simulink model "HW4_simulink"  (R2017b)
settings: Solver=VariableStepAuto  StartTime=0.0  StopTime=.167  RelTol=1e-3
values from neighbouring files (symbols this model uses):
  B = 0.8    [HW4_code.m]
  ia = 4    [HW4_code.m]
  l = 0.8    [HW4_code.m]
  r = 0.05    [HW4_code.m]
  w = 376.99    [HW4_code.m]
settings Model: Creator=Andrew McCullough  LastModifiedBy=Andrew McCullough

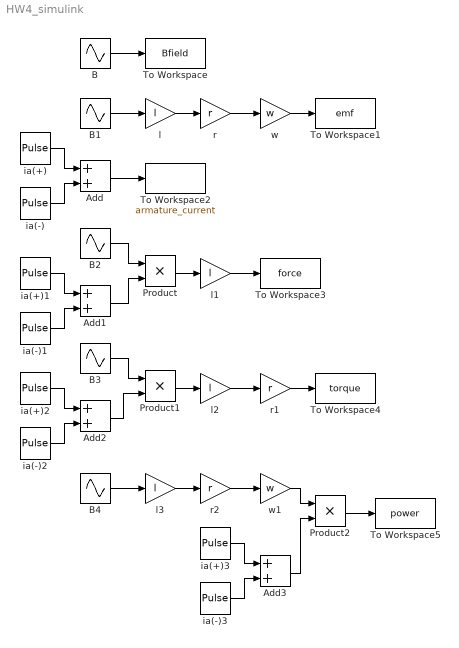
== system HW4_simulink ==
  Add{,1..3} (4 alike) : Sum
  B{,1..4} (5 alike) : Sin  Amplitude=B  Frequency=w  Phase=pi/2  SampleTime=.00001
  Product : Product
  Product1 : Product
  Product2 : Product
  To Workspace : ToWorkspace  VariableName=Bfield  SaveFormat=Timeseries  SampleTime=-1
  To Workspace1 : ToWorkspace  VariableName=emf  SaveFormat=Timeseries  SampleTime=-1
  To Workspace2 : ToWorkspace  VariableName=armature_current  SaveFormat=Timeseries  SampleTime=-1
  To Workspace3 : ToWorkspace  VariableName=force  SaveFormat=Timeseries  SampleTime=-1
  To Workspace4 : ToWorkspace  VariableName=torque  SaveFormat=Timeseries  SampleTime=-1
  To Workspace5 : ToWorkspace  VariableName=power  SaveFormat=Timeseries  SampleTime=-1
  ia(+){,1..3} (4 alike) : DiscretePulseGenerator  PulseType=Time based  Amplitude=ia  Period=.01667  PulseWidth=50  PhaseDelay=-.0041675
  ia(-){,1..3} (4 alike) : DiscretePulseGenerator  PulseType=Time based  Amplitude=-ia  Period=.01667  PulseWidth=50  PhaseDelay=.0041675
  l{,1..3} (4 alike) : Gain  Gain=l
  r : Gain  Gain=r
  r1 : Gain  Gain=r
  r2 : Gain  Gain=r
  w : Gain  Gain=w
  w1 : Gain  Gain=w
  wires:
  B1/1 -> l/1
  l/1 -> r/1
  r/1 -> w/1
  w/1 -> To Workspace1/1
  B/1 -> To Workspace/1
  Add/1 -> To Workspace2/1
  l1/1 -> To Workspace3/1
  Product/1 -> l1/1
  B2/1 -> Product/1
  Add1/1 -> Product/2
  Product1/1 -> l2/1
  Add2/1 -> Product1/2
  B3/1 -> Product1/1
  l2/1 -> r1/1
  r1/1 -> To Workspace4/1
  B4/1 -> l3/1
  r2/1 -> w1/1
  l3/1 -> r2/1
  w1/1 -> Product2/1
  Add3/1 -> Product2/2
  Product2/1 -> To Workspace5/1
  ia(+)/1 -> Add/1
  ia(-)/1 -> Add/2
  ia(+)1/1 -> Add1/1
  ia(-)1/1 -> Add1/2
  ia(+)2/1 -> Add2/1
  ia(-)2/1 -> Add2/2
  ia(+)3/1 -> Add3/1
  ia(-)3/1 -> Add3/2
